simulink model "TP3_MinSeg_SBR"  (R2021b)
settings: Solver=FixedStepDiscrete  StartTime=0.0  StopTime=10  FixedStep=.03  RelTol=1e-3  EnableMultiTasking=on
PostLoadFcn:
  | try,
  | codertarget.arduinobase.registry.setBaudRate(gcs,115200)
  | disp('baud rate set to 115200 for external mode hardware serial')
  | baudrate='set_to_115200'
  | catch
  | disp('baud rate setting not needed in this version')
  | end
values from neighbouring files (symbols this model uses):
  EncCov = 2*pi/1336    (= 0.00470298301436)    [script.m]
  GyroRad = pi*4.2386E-5    (= 0.000133159546215)    [script.m]
  h = 0.03    [script.m]
  L2 = L1.*[1 1 Rw Rw]    [script.m]
undefined symbols (not defined in the file or in its folder): DiscIntNeverNeededParam
libraries: RASPlib x4, MinSegLibrary_M2V5 x3, simulink x2
settings Model: SimulationMode=external  ExtModeTrigDuration=2  Creator=Alec  LastModifiedBy=Dylan
settings SolverCC: AlgebraicLoopSolver=TrustRegion
settings DataIOCC: LimitDataPoints=on  SaveFormat=Array  ReturnWorkspaceOutputs=off
settings OptimizationCC: EnhancedBackFolding=on  PassReuseOutputArgsThreshold=0  ExpressionDepthLimit=2147483647  MaxStackSize=64  OptimizeBlockOrder=speed  DifferentSizesBufferReuse=on  OptimizationCustomize=off
settings DebuggingCC: UnderspecifiedInitializationDetection=Classic  MergeDetectMultiDrivingBlocksExec=none  ParameterTunabilityLossMsg=error  StateNameClashWarn=warning  SFUnexpectedBacktrackingDiag=warning  SFNoUnconditionalDefaultTransitionDiag=warning  SFExecutionAtInitializationDiag=none  SFMachineParentedDataDiag=warning  ArithmeticOperatorsInVariantConditions=warning
settings HardwareCC: ProdBitPerInt=16  ProdBitPerPointer=16  ProdBitPerSizeT=16  ProdBitPerPtrDiffT=16  ProdLargestAtomicFloat=None  ProdWordSize=8  ProdHWDeviceType=Atmel->AVR  UseEmbeddedCoderFeatures=off  UseSimulinkCoderFeatures=off
settings ModelReferenceCC: PropagateSignalLabelsOutOfModel=off
settings SFSimCC: SimUseLocalCustomCode=off  MATLABDynamicMemAlloc=off  CustomCodeUndefinedFunction=UseInterfaceOnly
settings RTWCC: Description=Embedded Coder  SystemTargetFile=ert.tlc  HardwareBoard=Arduino Mega 2560  TemplateMakefile=ert_default_tmf  GenerateReport=on  RTWVerbose=off  RTWUseLocalCustomCode=off  Toolchain=Arduino AVR  BuildConfiguration=Faster Runs  LaunchReport=on
settings CodeAppCC: ForceParamTrailComments=on  OperatorAnnotations=on  MangleLength=10
settings ERTTargetCC: ERTCustomFileBanners=off  SupportContinuousTime=on  SupportNonInlinedSFcns=on  RemoveResetFunc=off  SupportVariableSizeSignals=on  ModelStepFunctionPrototypeControlCompliant=off  ExtModeStaticAllocSize=2048
settings ConfigComp: CovMetricSettings=dw  CovSaveCumulativeToWorkspaceVar=on  CovSaveSingleToWorkspaceVar=on  CovExternalEMLEnable=off

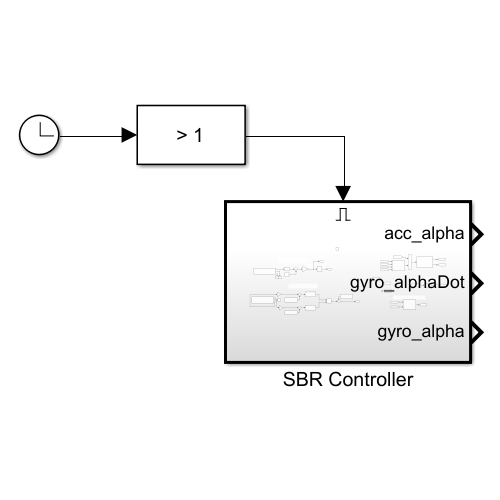
[thumbnail: Simulink's stored preview of the top-level diagram]
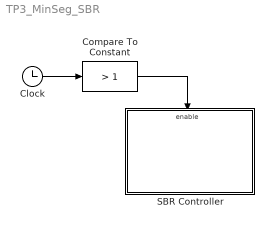
== system TP3_MinSeg_SBR ==
  Clock : Clock
  Compare To Constant : simulink/Logic and Bit Operations/Compare To Constant  relop=>  const=1  OutDataTypeStr=boolean
  SBR Controller : Subsystem
  wires:
  Compare To Constant/1 -> SBR Controller/Enable
  Clock/1 -> Compare To Constant/1

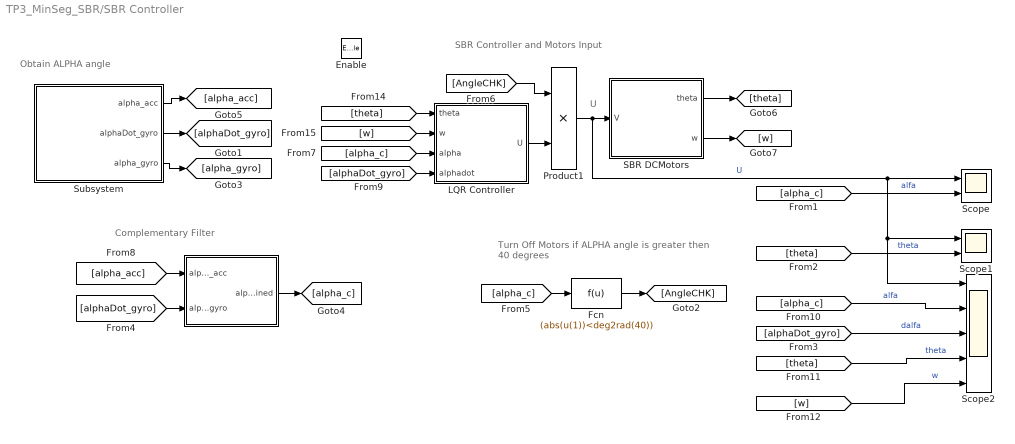
== system TP3_MinSeg_SBR/SBR Controller ==
  note: Complementary Filter
  note: Turn Off Motors if ALPHA angle
      | is greater then 40 degrees
  note: U
  note: Obtain ALPHA angle
  note: SBR Controller and Motors Input
  Enable : EnablePort
  " " : Subsystem
  Fcn : Fcn  Expr=(abs(u(1))<deg2rad(40))
  LQR Controller : Subsystem
  Product1 : Product  RndMeth=Zero
  SBR DCMotors : Subsystem
  Scope : Scope  NumInputPorts=2
  Scope1 : Scope  NumInputPorts=2
  Scope2 : Scope  NumInputPorts=5
  Subsystem : Subsystem
  wires:
  " "/1(alpha_combined) -> [alpha_c]
  [alphaDot_gyro] -> " "/2(alphaDot_gyro)
  [alpha_acc] -> " "/1(alpha_acc)
  Fcn/1 -> [AngleCHK]
  [alpha_c] -> Fcn/1
  [AngleCHK] -> Product1/1
  Product1/1 -> Scope2/1, Scope1/1, Scope/1, SBR DCMotors/1(V)  "U"
  SBR DCMotors/2(w) -> [w]
  SBR DCMotors/1(theta) -> [theta]
  [theta] -> LQR Controller/1(theta)
  [w] -> LQR Controller/2(w)
  [alpha_c] -> LQR Controller/3(alpha)
  [alphaDot_gyro] -> LQR Controller/4(alphadot)
  LQR Controller/1(U) -> Product1/2
  Subsystem/2(alphaDot_gyro) -> [alphaDot_gyro]
  Subsystem/1(alpha_acc) -> [alpha_acc]
  Subsystem/3(alpha_gyro) -> [alpha_gyro]
  [alpha_c] -> Scope/2  "alfa"
  [theta] -> Scope1/2  "theta"
  [alphaDot_gyro] -> Scope2/3  "dalfa"
  [alpha_c] -> Scope2/2  "alfa"
  [theta] -> Scope2/4  "theta"
  [w] -> Scope2/5  "w"

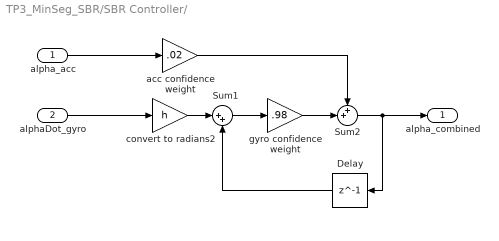
== system TP3_MinSeg_SBR/SBR Controller/  ==
  alpha_acc : Inport
  alphaDot_gyro : Inport  Port=2
  Delay : Delay  DelayLength=1  SampleTime=h
  Sum1 : Sum  Inputs=|++
  Sum2 : Sum  Inputs=++|
  acc confidence weight : Gain  Gain=.02  OutDataTypeStr=single
  convert to radians2 : Gain  Gain=h  OutDataTypeStr=single
  gyro confidence weight : Gain  Gain=.98  OutDataTypeStr=single
  alpha_combined : Outport
  wires:
  alphaDot_gyro/1 -> convert to radians2/1
  Sum1/1 -> gyro confidence weight/1
  acc confidence weight/1 -> Sum2/1
  alpha_acc/1 -> acc confidence weight/1
  gyro confidence weight/1 -> Sum2/2
  Delay/1 -> Sum1/2
  convert to radians2/1 -> Sum1/1
  Sum2/1 -> Delay/1, alpha_combined/1

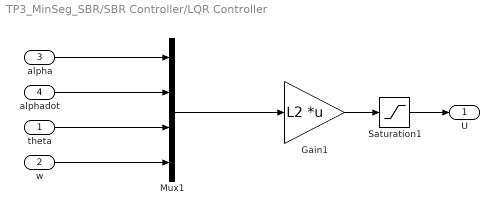
== system TP3_MinSeg_SBR/SBR Controller/LQR Controller ==
  theta : Inport
  w : Inport  Port=2
  alpha : Inport  Port=3
  alphadot : Inport  Port=4
  Gain1 : Gain  Gain=L2  Multiplication=Matrix(K*u) (u vector)
  Mux1 : Mux
  Saturation1 : Saturate  UpperLimit=4.8  LowerLimit=-4.8
  U : Outport
  wires:
  Mux1/1 -> Gain1/1
  Gain1/1 -> Saturation1/1
  Saturation1/1 -> U/1
  alpha/1 -> Mux1/1
  alphadot/1 -> Mux1/2
  theta/1 -> Mux1/3
  w/1 -> Mux1/4

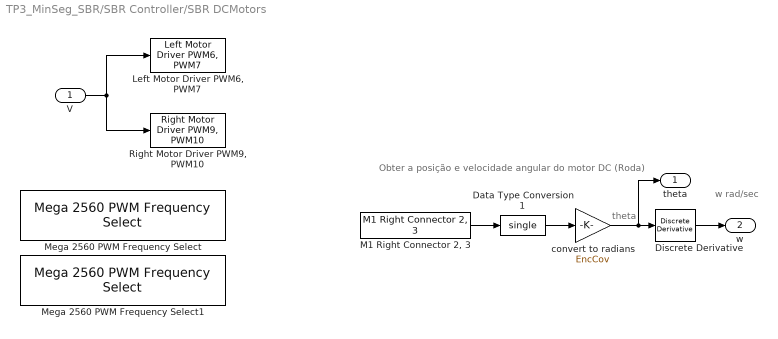
== system TP3_MinSeg_SBR/SBR Controller/SBR DCMotors ==
  note: Obter a posição e velocidade angular do motor DC (Roda)
  note: w
      | rad/sec
  note: theta
  V : Inport
  Data Type Conversion1 : DataTypeConversion  OutDataTypeStr=single
  Discrete Derivative : simulink/Discrete/Discrete Derivative  gainval=1.0  ICPrevScaledInput=0.0  OutMin=[]  OutMax=[]  OutDataType=fixdt(1, 16)  OutScaling=2^-10  DoSatur=off
  "Left Motor Driver PWM6, PWM7" : MinSegLibrary_M2V5/Left Motor Driver PWM6, PWM7  Vsupply=4.8  PWMoffset=0
      settings: SourceProductName=Rensselaer Arduino Support Package
  "M1 Right Connector 2, 3" : MinSegLibrary_M2V5/M1 Right Connector 2, 3  Encoder=0  PinA=2  PinB=3
      settings: SourceProductName=Rensselaer Arduino Support Package
  Mega 2560 PWM Frequency Select : RASPlib/Mega 2560 PWM Frequency Select  Frequency=32KHz  Timer=4 - pins 6, 7, 8
      settings: SourceProductName=Rensselaer Arduino Support Package
  Mega 2560 PWM Frequency Select1 : RASPlib/Mega 2560 PWM Frequency Select  Frequency=32KHz  Timer=2 - pins 9, 10
      settings: SourceProductName=Rensselaer Arduino Support Package
  "Right Motor Driver PWM9, PWM10 " : MinSegLibrary_M2V5/Right Motor Driver PWM9, PWM10   Vsupply=4.8  PWMoffset=0
      settings: SourceProductName=Rensselaer Arduino Support Package
  convert to radians : Gain  Gain=EncCov  OutDataTypeStr=single
  theta : Outport
  w : Outport  Port=2
  wires:
  Data Type Conversion1/1 -> convert to radians/1
  convert to radians/1 -> theta/1, Discrete Derivative/1
  V/1 -> "Left Motor Driver PWM6, PWM7"/1, "Right Motor Driver PWM9, PWM10 "/1
  "M1 Right Connector 2, 3"/1 -> Data Type Conversion1/1
  Discrete Derivative/1 -> w/1

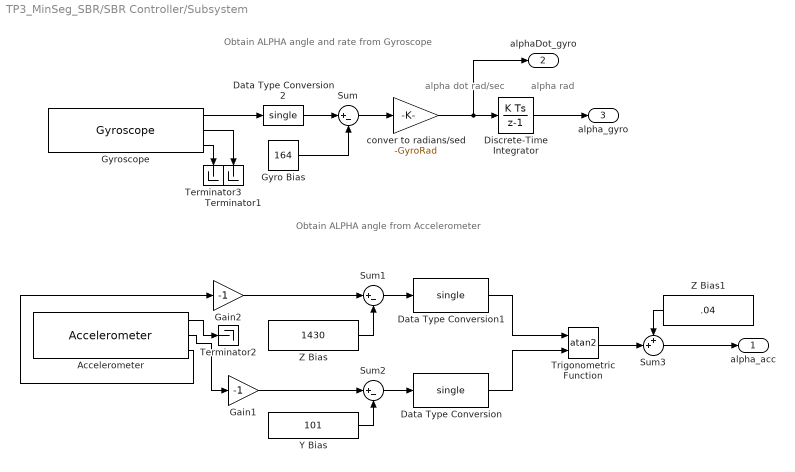
== system TP3_MinSeg_SBR/SBR Controller/Subsystem ==
  note: alpha
      | rad
  note: Obtain ALPHA angle and rate from Gyroscope
  note: alpha dot
      | rad/sec
  note: Obtain ALPHA angle from Accelerometer
  "Accelerometer " : RASPlib/Accelerometer  SimulateUsing=Code generation
      settings: SourceProductName=Rensselaer Arduino Support Package
  Data Type Conversion2 : DataTypeConversion  OutDataTypeStr=single
  Data Type Conversion : DataTypeConversion  OutDataTypeStr=single
  Data Type Conversion1 : DataTypeConversion  OutDataTypeStr=single
  Discrete-Time Integrator : DiscreteIntegrator  SampleTime=h  ICPrevOutput=DiscIntNeverNeededParam  ICPrevScaledInput=DiscIntNeverNeededParam
  Gain1 : Gain  Gain=-1
  Gain2 : Gain  Gain=-1
  Gyro Bias : Constant  Value=164  SampleTime=h
  "Gyroscope " : RASPlib/Gyroscope  DLPFmode=0
      settings: SourceProductName=Rensselaer Arduino Support Package
  Sum : Sum  Inputs=|+-
  Sum1 : Sum  Inputs=|+-
  Sum2 : Sum  Inputs=|+-
  Sum3 : Sum  Inputs=++|
  Terminator1 : Terminator
  Terminator2 : Terminator
  Terminator3 : Terminator
  Trigonometric Function : Trigonometry  Operator=atan2
  Y Bias : Constant  Value=101
  Z Bias : Constant  Value=1430
  Z Bias1 : Constant  Value=.04  OutDataTypeStr=single
  conver to radians/sed : Gain  Gain=-GyroRad  OutDataTypeStr=single
  alpha_acc : Outport
  alphaDot_gyro : Outport  Port=2
  alpha_gyro : Outport  Port=3
  wires:
  Sum1/1 -> Data Type Conversion1/1
  Gain2/1 -> Sum1/1
  Trigonometric Function/1 -> Sum3/2
  Gyro Bias/1 -> Sum/2
  Gain1/1 -> Sum2/1
  Data Type Conversion2/1 -> Sum/1
  Data Type Conversion/1 -> Trigonometric Function/2
  conver to radians/sed/1 -> alphaDot_gyro/1, Discrete-Time Integrator/1
  "Accelerometer "/1 -> Terminator2/1
  Y Bias/1 -> Sum2/2
  Sum3/1 -> alpha_acc/1
  Sum/1 -> conver to radians/sed/1
  Z Bias/1 -> Sum1/2
  Data Type Conversion1/1 -> Trigonometric Function/1
  Z Bias1/1 -> Sum3/1
  "Gyroscope "/3 -> Terminator3/1
  Sum2/1 -> Data Type Conversion/1
  "Gyroscope "/1 -> Data Type Conversion2/1
  "Accelerometer "/2 -> Gain1/1
  Discrete-Time Integrator/1 -> alpha_gyro/1
  "Accelerometer "/3 -> Gain2/1
  "Gyroscope "/2 -> Terminator1/1
